simulink library "lib_contact_model"  (Simulink 8.5)
settings: Solver=ode45  StartTime=0.0  StopTime=10.0  RelTol=1e-3
undefined symbols (not defined in the file or in its folder): HC_params
undefined symbols (not defined in the file): HC_q_max, HC_q_min
settings Model: Creator=schappler  LastModifiedBy=schappler

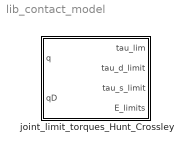
== system lib_contact_model ==
  joint_limit_torques_Hunt_Crossley : Subsystem  mask{HC_params=HC_params, q_min=HC_q_min, q_max=HC_q_max}
      mask prompts: HC_params "Parameter des Hunt-Crossley-Modells (R, h, alpha)"

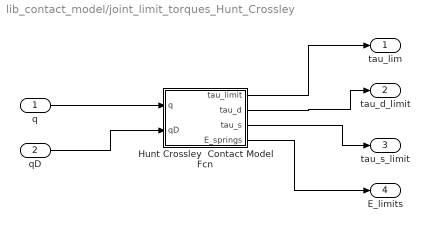
== system lib_contact_model/joint_limit_torques_Hunt_Crossley ==
  q : Inport
  qD : Inport  Port=2
  Hunt Crossley  Contact Model Fcn : MATLAB Function  TreatAsAtomicUnit=on
  tau_lim : Outport
  tau_d_limit : Outport  Port=2
  tau_s_limit : Outport  Port=3
  E_limits : Outport  Port=4
  wires:
  Hunt Crossley  Contact Model Fcn/4(E_springs) -> E_limits/1
  Hunt Crossley  Contact Model Fcn/1(tau_limit) -> tau_lim/1
  Hunt Crossley  Contact Model Fcn/3(tau_s) -> tau_s_limit/1
  Hunt Crossley  Contact Model Fcn/2(tau_d) -> tau_d_limit/1
  q/1 -> Hunt Crossley  Contact Model Fcn/1(q)
  qD/1 -> Hunt Crossley  Contact Model Fcn/2(qD)

== matlab function joint_limit_torques_Hunt_Crossley/Hunt Crossley Contact Model Fcn ==
  data: q input double; qD input double; tau_limit output double; HC_params parameter double; tau_d output double; tau_s output double; q_min parameter double; q_max parameter double; E_springs output double
function [tau_limit,tau_d,tau_s,E_springs]= fcn(q,qD,HC_params, q_min, q_max)
%#codegen

[tau_s,tau_d,E_springs]=joint_limit_torques_Hunt_Crossley(q,qD,HC_params, q_min, q_max);
tau_limit=tau_s+tau_d;
